simulink model "DCmotor_Speed_Ctrl"  (R2021b)
settings: Solver=FixedStepAuto  StartTime=0.0  StopTime=inf  FixedStep=Ts  RelTol=1e-3  EnableMultiTasking=on
values from neighbouring files (symbols this model uses):
  den_Gd = Gd.Den{:}    [para.m]
  encoder_scale = 1/12/4 *2*pi    (= 0.1308996939)    [para.m]
  Ki = 50    [para.m]
  Kp = 100    [para.m]
  num_Gd = Gd.Num{:}    [para.m]
  Ts = 1e-2    (= 0.01)    [para.m]
  Vlim = 12    [para.m]
  Wref = 100    [para.m]
libraries: arduinolib x1, simulink x1, arduinosensorlib x1
settings Model: ExtModeBatchMode=on  ExtModeTrigDuration=2  Creator=user  LastModifiedBy=user
settings OptimizationCC: EnhancedBackFolding=on  PassReuseOutputArgsAs=Individual arguments  ZeroExternalMemoryAtStartup=off  ZeroInternalMemoryAtStartup=off  MaxStackSize=64  OptimizeBlockOrder=speed  DifferentSizesBufferReuse=on  OptimizationCustomize=off  EfficientTunableParamExpr=on
settings DebuggingCC: ParameterTunabilityLossMsg=error
settings HardwareCC: ProdBitPerInt=16  ProdBitPerPointer=16  ProdBitPerSizeT=16  ProdBitPerPtrDiffT=16  ProdLargestAtomicFloat=None  ProdWordSize=8  ProdHWDeviceType=Atmel->AVR
settings SFSimCC: MATLABDynamicMemAlloc=off
settings RTWCC: Description=Embedded Coder  SystemTargetFile=ert.tlc  HardwareBoard=Arduino Mega 2560  TemplateMakefile=ert_default_tmf  Toolchain=Arduino AVR  BuildConfiguration=Faster Runs
settings CodeAppCC: ForceParamTrailComments=on  IgnoreCustomStorageClasses=off  OperatorAnnotations=on  SimulinkDataObjDesc=on  SFDataObjDesc=on  InsertBlockDesc=on
settings ERTTargetCC: SupportContinuousTime=on  SupportVariableSizeSignals=on  ExtModeTransport=3  ExtModeStaticAlloc=on  ExtModeStaticAllocSize=2048  ExtModeMexFile=ext_xcp  ExtModeIntrfLevel=Level2 - Open

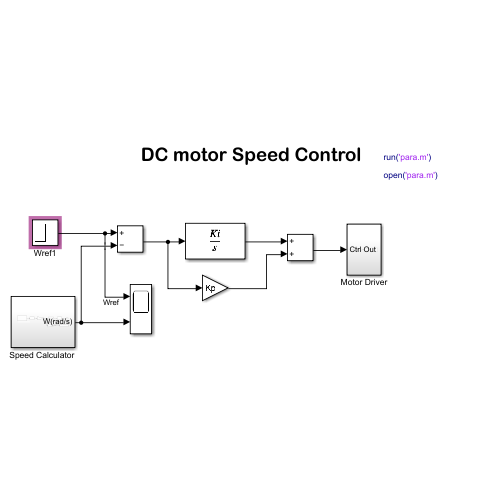
[thumbnail: Simulink's stored preview of the top-level diagram]
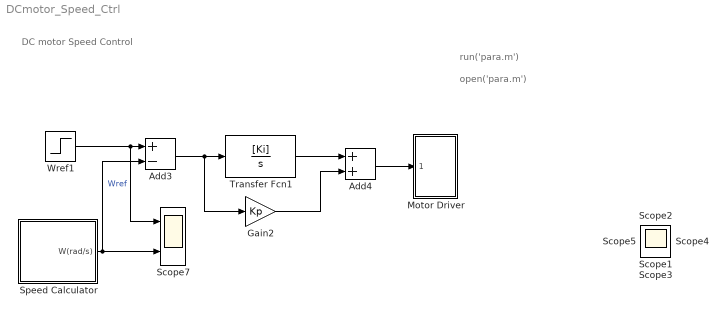
== system DCmotor_Speed_Ctrl ==
  note: open('para.m')
  note: run('para.m')
  note: DC motor Speed Control
  Add3 : Sum  Inputs=+-
  Add4 : Sum
  Gain2 : Gain  Gain=Kp
  Motor Driver : Subsystem
  Scope7 : Scope  NumInputPorts=2
  "Speed Calculator " : Subsystem
  Transfer Fcn1 : TransferFcn  Numerator=[Ki]  Denominator=[1 0]
  Wref1 : Step  Time=0  After=Wref  SampleTime=0
  Scope{1..5} (5 alike) : Scope
  wires:
  Transfer Fcn1/1 -> Add4/1
  Add3/1 -> Gain2/1, Transfer Fcn1/1
  Wref1/1 -> Scope7/1, Add3/1  "Wref"
  Gain2/1 -> Add4/2
  "Speed Calculator "/1(W(rad/s)) -> Scope7/2, Add3/2
  Add4/1 -> Motor Driver/1(Ctrl Out)

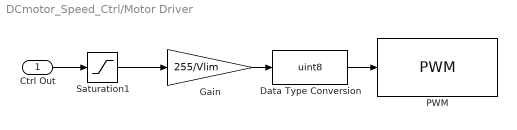
== system DCmotor_Speed_Ctrl/Motor Driver ==
  Ctrl Out : Inport
  Data Type Conversion : DataTypeConversion  OutDataTypeStr=uint8
  Gain : Gain  Gain=255/Vlim
  PWM : arduinolib/PWM  pinNumber=11  frequencyType=Default  desiredFrequency=490.2  achievableFrequency=490.2
  Saturation1 : Saturate  UpperLimit=Vlim  LowerLimit=0
  wires:
  Saturation1/1 -> Gain/1
  Gain/1 -> Data Type Conversion/1
  Data Type Conversion/1 -> PWM/1
  Ctrl Out/1 -> Saturation1/1

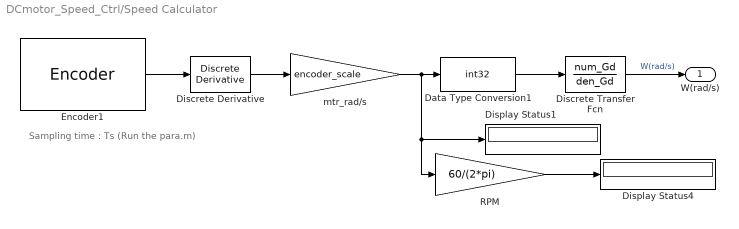
== system DCmotor_Speed_Ctrl/Speed Calculator  ==
  note: Sampling time : Ts (Run the para.m)
  Data Type Conversion1 : DataTypeConversion  OutDataTypeStr=int32
  Discrete Transfer Fcn : DiscreteTransferFcn  Numerator=num_Gd  Denominator=den_Gd  SampleTime=Ts
  Discrete Derivative : simulink/Discrete/Discrete Derivative  gainval=1  ICPrevScaledInput=0.0  OutMin=[]  OutMax=[]  OutDataType=fixdt(1, 16)  OutScaling=2^-10  DoSatur=off
  Display Status1 : Display
  Display Status4 : Display
  Encoder1 : arduinosensorlib/Encoder  InputA=18  InputB=19  Mode=No reset  SampleTime=Ts
      settings: SourceProductBaseCode=ARDUINO
  RPM : Gain  Gain=60/(2*pi)
  mtr_rad/s : Gain  Gain=encoder_scale
  W(rad/s) : Outport
  wires:
  Data Type Conversion1/1 -> Discrete Transfer Fcn/1
  mtr_rad/s/1 -> Data Type Conversion1/1, RPM/1, Display Status1/1
  RPM/1 -> Display Status4/1
  Encoder1/1 -> Discrete Derivative/1
  Discrete Derivative/1 -> mtr_rad/s/1
  Discrete Transfer Fcn/1 -> W(rad/s)/1  "W(rad/s)"
